simulink model "pm_id_model_PI_anti_windup"  (R2022b)
settings: Solver=VariableStepAuto  StartTime=0.0  StopTime=2  MaxStep=0.0005  RelTol=1e-3
undefined symbols (not defined in the file): Ld, Rs
libraries: slpidlib x1
settings Model: Creator=jack  LastModifiedBy=jack

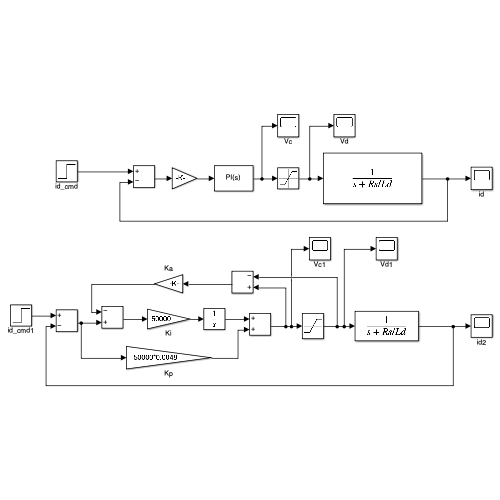
[thumbnail: Simulink's stored preview of the top-level diagram]
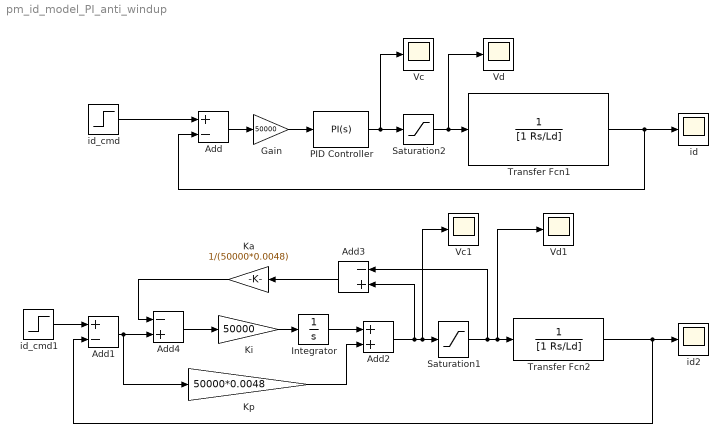
== system pm_id_model_PI_anti_windup ==
  Add : Sum  Inputs=+-
  Add1 : Sum  Inputs=+-
  Add2 : Sum
  Add3 : Sum  Inputs=-+
  Add4 : Sum  Inputs=-+
  Gain : Gain  Gain=50000
  Integrator : Integrator
  Ka : Gain  Gain=1/(50000*0.0048)
  Ki : Gain  Gain=50000
  Kp : Gain  Gain=50000*0.0048
  PID Controller : slpidlib/PID Controller  Controller=PI  Form=Parallel  TimeDomain=Continuous-time  UseExternalTs=off  SampleTime=-1  IntegratorMethod=Forward Euler  FilterMethod=Forward Euler  ControllerParametersSource=internal  P=0.0048  I=1  UseKiTs=off  D=0  N=100  UseFilter=on  TunerSelectOption=Transfer Function Based (PID Tuner App)  InitialConditionSource=internal  InitialConditionForIntegrator=0  InitialConditionForFilter=0  DifferentiatorICPrevScaledInput=0  ExternalReset=none  TrackingMode=off  Kt=1  LimitOutput=off  SatLimitsSource=internal  UpperSaturationLimit=inf  LowerSaturationLimit=-inf  LinearizeAsGain=on  AntiWindupMode=none  Kb=1  LimitIntegrator=off  UpperIntegratorSaturationLimit=inf  LowerIntegratorSaturationLimit=-inf  POutMin=[]  POutMax=[]  IOutMin=[]  IOutMax=[]  DOutMin=[]  DOutMax=[]  NOutMin=[]  NOutMax=[]  SumOutMin=[]  SumOutMax=[]  SaturationOutMin=[]  SaturationOutMax=[]  PParamMin=[]  PParamMax=[]  IParamMin=[]  IParamMax=[]  DParamMin=[]  DParamMax=[]  NParamMin=[]  NParamMax=[]  KbParamMin=[]  KbParamMax=[]  KtParamMin=[]  KtParamMax=[]  KbOutMin=[]  KbOutMax=[]  KtOutMin=[]  KtOutMax=[]  IntegratorOutMin=[]  IntegratorOutMax=[]  FilterOutMin=[]  FilterOutMax=[]  SumI1OutMin=[]  SumI1OutMax=[]  SumI2OutMin=[]  SumI2OutMax=[]  SumI3OutMin=[]  SumI3OutMax=[]  SumI4OutMin=[]  SumI4OutMax=[]  SumDOutMin=[]  SumDOutMax=[]  DifferentiatorOutMin=[]  DifferentiatorOutMax=[]  FilterDiffOutCoefMin=[]  FilterDiffOutCoefMax=[]  ReciprocalOutMin=[]  ReciprocalOutMax=[]  SumDenOutMin=[]  SumDenOutMax=[]  SumNumOutMin=[]  SumNumOutMax=[]  DivideOutMin=[]  DivideOutMax=[]  UdiffTsProdOutMin=[]  UdiffTsProdOutMax=[]  NTsProdOutMin=[]  NTsProdOutMax=[]  UintegralTsProdOutMin=[]  UintegralTsProdOutMax=[]  UngainTsProdOutMin=[]  UngainTsProdOutMax=[]  ClampingZeroOutDataTypeStr=Inherit: Inherit via back propagation  ClampingZeroOutMin=[]  ClampingZeroOutMax=[]  FilterDenConstantOutDataTypeStr=Inherit: Inherit via back propagation  FilterDenConstantOutMin=[]  FilterDenConstantOutMax=[]  PCopyOutDataTypeStr=Inherit: Inherit via back propagation  PCopyOutMin=[]  PCopyOutMax=[]  NCopyOutDataTypeStr=Inherit: Inherit via back propagation  NCopyOutMin=[]  NCopyOutMax=[]  IntegratorContinuousStateAttributes=''  IntegratorStateMustResolveToSignalObject=off  IntegratorRTWStateStorageClass=Auto  FilterContinuousStateAttributes=''  FilterStateMustResolveToSignalObject=off  FilterRTWStateStorageClass=Auto  ParallelPVariant=InternalParameters  IdealPVariant=Disabled  IVariant=InternalParameters  DVariant=Disabled  IntegratorVariant=Continuous  SatVariant=Disabled  AWVariant=Passthrough  PCopyVariant=Disabled  TRVariant=Disabled  FdbkBlocksVariant=Forward  IdealPFdbkVariant=Disabled  SatFdbkVariant=Disabled  DerivativeFilterVariant=Disabled  NVariant=Disabled  NCopyVariant=Disabled_SignalSpec  FilterICVariant=Disabled  IntegratorICVariant=InternalICs  ExternalResetVariant=Disabled  TRSumVariant=Passthrough  SumFdbkVariant=Disabled  SumVariant=Sum_PI  TsampFilterVariant=InternalTs  TsampNgainVariant=Passthrough  TsampIntegralVariant=Passthrough  ExternalSaturationOutDataTypeStr=Inherit: Same as second input
  Saturation1 : Saturate  UpperLimit=150  LowerLimit=-150
  Saturation2 : Saturate  UpperLimit=150  LowerLimit=-150
  Transfer Fcn1 : TransferFcn  Denominator=[1 Rs/Ld]
  Transfer Fcn2 : TransferFcn  Denominator=[1 Rs/Ld]
  Vc : Scope
  Vc1 : Scope
  Vd : Scope
  Vd1 : Scope
  id : Scope
  id2 : Scope
  id_cmd : Step  SampleTime=0
  id_cmd1 : Step  SampleTime=0
  wires:
  Transfer Fcn1/1 -> id/1, Add/2
  id_cmd/1 -> Add/1
  Add/1 -> Gain/1
  Gain/1 -> PID Controller/1
  PID Controller/1 -> Vc/1, Saturation2/1
  Saturation1/1 -> Add3/1, Vd1/1, Transfer Fcn2/1
  Ki/1 -> Integrator/1
  id_cmd1/1 -> Add1/1
  Transfer Fcn2/1 -> Add1/2, id2/1
  Integrator/1 -> Add2/1
  Kp/1 -> Add2/2
  Add2/1 -> Add3/2, Vc1/1, Saturation1/1
  Add3/1 -> Ka/1
  Add1/1 -> Kp/1, Add4/2
  Ka/1 -> Add4/1
  Add4/1 -> Ki/1
  Saturation2/1 -> Transfer Fcn1/1, Vd/1
